simulink model "Simulink_Library_Example"  (R2021b)
settings: Solver=VariableStepAuto  StartTime=0.0  StopTime=10.0  RelTol=1e-3
libraries: Simulink_Library_Example_Lib x3
settings Model: Creator=waleed.elshemy  LastModifiedBy=waleed.elshemy

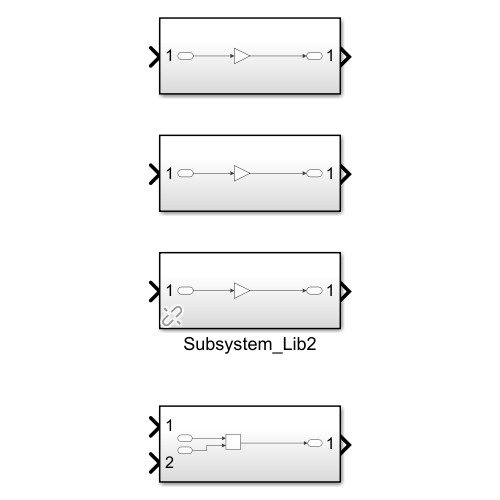
[thumbnail: Simulink's stored preview of the top-level diagram]
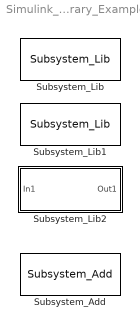
== system Simulink_Library_Example ==
  Subsystem_Add : Simulink_Library_Example_Lib/Subsystem_Add  SystemSampleTime=-1  VariantActivationTime=update diagram  Latency=0  AutoFrameSizeCalculation=off
  Subsystem_Lib : Simulink_Library_Example_Lib/Subsystem_Lib  SystemSampleTime=-1  VariantActivationTime=update diagram  Latency=0  AutoFrameSizeCalculation=off
  Subsystem_Lib1 : Simulink_Library_Example_Lib/Subsystem_Lib  SystemSampleTime=-1  VariantActivationTime=update diagram  Latency=0  AutoFrameSizeCalculation=off
  Subsystem_Lib2 : Subsystem  AncestorBlock=Simulink_Library_Example_Lib/Subsystem_Lib

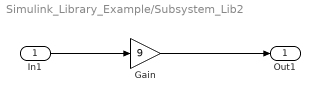
== system Simulink_Library_Example/Subsystem_Lib2 ==
  In1 : Inport
  Gain : Gain  Gain=9
  Out1 : Outport
  wires:
  Gain/1 -> Out1/1
  In1/1 -> Gain/1
